simulink model "EvaluasiHIV"  (R2020a)
settings: Solver=VariableStepAuto  StartTime=0.0  StopTime=1  RelTol=1e-3
settings Model: Creator=armel  LastModifiedBy=Anwar

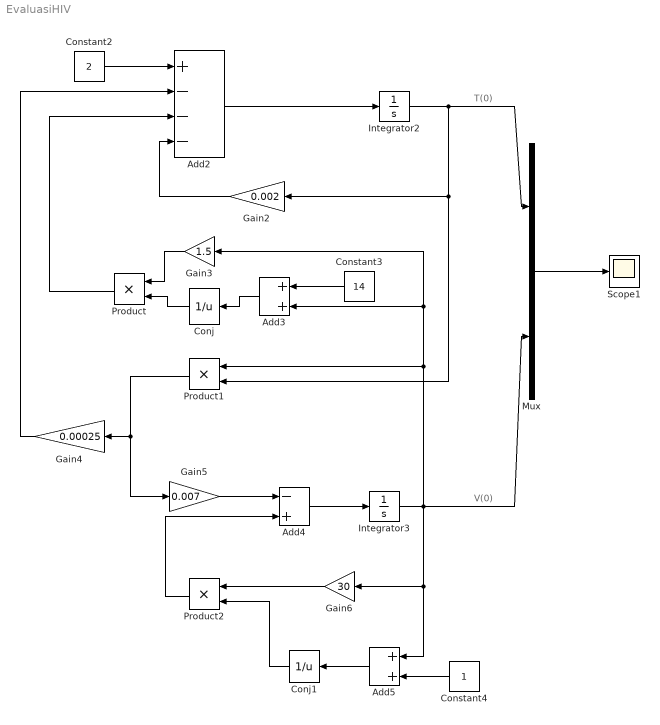
== system EvaluasiHIV ==
  note: V(0)
  note: T(0)
  Add2 : Sum  Inputs=+---
  Add3 : Sum
  Add4 : Sum  Inputs=-+
  Add5 : Sum
  Conj : Math  Operator=reciprocal  SaturateOnIntegerOverflow=on
  Conj1 : Math  Operator=reciprocal  SaturateOnIntegerOverflow=on
  Constant2 : Constant  Value=2
  Constant3 : Constant  Value=14
  Constant4 : Constant
  Gain2 : Gain  Gain=0.002
  Gain3 : Gain  Gain=1.5
  Gain4 : Gain  Gain=0.00025
  Gain5 : Gain  Gain=0.007
  Gain6 : Gain  Gain=30
  Integrator2 : Integrator  InitialCondition=1000
  Integrator3 : Integrator  InitialCondition=1000
  Mux : Mux  Inputs=2
  Product : Product
  Product1 : Product
  Product2 : Product
  Scope1 : Scope
  wires:
  Constant2/1 -> Add2/1
  Add2/1 -> Integrator2/1
  Integrator2/1 -> Product1/2, Gain2/1, Mux/1
  Gain2/1 -> Add2/4
  Constant3/1 -> Add3/1
  Gain3/1 -> Product/1
  Product/1 -> Add2/3
  Add3/1 -> Conj/1
  Conj/1 -> Product/2
  Product1/1 -> Gain5/1, Gain4/1
  Gain4/1 -> Add2/2
  Gain5/1 -> Add4/1
  Add4/1 -> Integrator3/1
  Integrator3/1 -> Gain3/1, Add3/2, Product1/1, Mux/2, Gain6/1, Add5/1
  Gain6/1 -> Product2/1
  Product2/1 -> Add4/2
  Conj1/1 -> Product2/2
  Add5/1 -> Conj1/1
  Constant4/1 -> Add5/2
  Mux/1 -> Scope1/1
